simulink model "Dc_motor_Rpi"  (R2019a)
settings: Solver=FixedStepAuto  StartTime=0.0  StopTime=inf  FixedStep=0.02  RelTol=1e-3  EnableMultiTasking=on
libraries: embdlinuxlib x2, raspberrypilib x2
settings Model: SimulationMode=external  Creator=Ghofrane  LastModifiedBy=Ghofrane
settings SolverCC: PositivePriorityOrder=on
settings OptimizationCC: EnhancedBackFolding=on  PassReuseOutputArgsAs=Individual arguments  MaxStackSize=64  OptimizeBlockOrder=speed  DifferentSizesBufferReuse=on  OptimizationCustomize=off
settings DebuggingCC: ParameterTunabilityLossMsg=error
settings HardwareCC: ProdBitPerPointer=32  ProdBitPerSizeT=32  ProdBitPerPtrDiffT=32  ProdLargestAtomicInteger=Long  ProdLargestAtomicFloat=Double  ProdWordSize=32  ProdLongLongMode=on  ProdHWDeviceType=ARM Compatible->ARM Cortex
settings SFSimCC: MATLABDynamicMemAlloc=off
settings RTWCC: SystemTargetFile=ert.tlc  HardwareBoard=Raspberry Pi  TLCOptions="-aInlineSetEventsForThisBaseRateFcn=TLC_FALSE -aSuppressMultiTaskScheduler=TLC_FALSE  -aRateBasedStepFcn=0"  TemplateMakefile=ert_default_tmf  GenerateReport=on  Toolchain=GNU GCC Raspberry Pi  BuildConfiguration=Faster Runs  IncludeHyperlinkInReport=on  LaunchReport=on  GenerateTraceInfo=on  GenerateTraceReport=on  GenerateTraceReportSl=on  GenerateTraceReportSf=on  GenerateTraceReportEml=on
settings CodeAppCC: ForceParamTrailComments=on  IgnoreCustomStorageClasses=off  OperatorAnnotations=on  SimulinkDataObjDesc=on  SFDataObjDesc=on  InsertBlockDesc=on
settings ERTTargetCC: SupportVariableSizeSignals=on

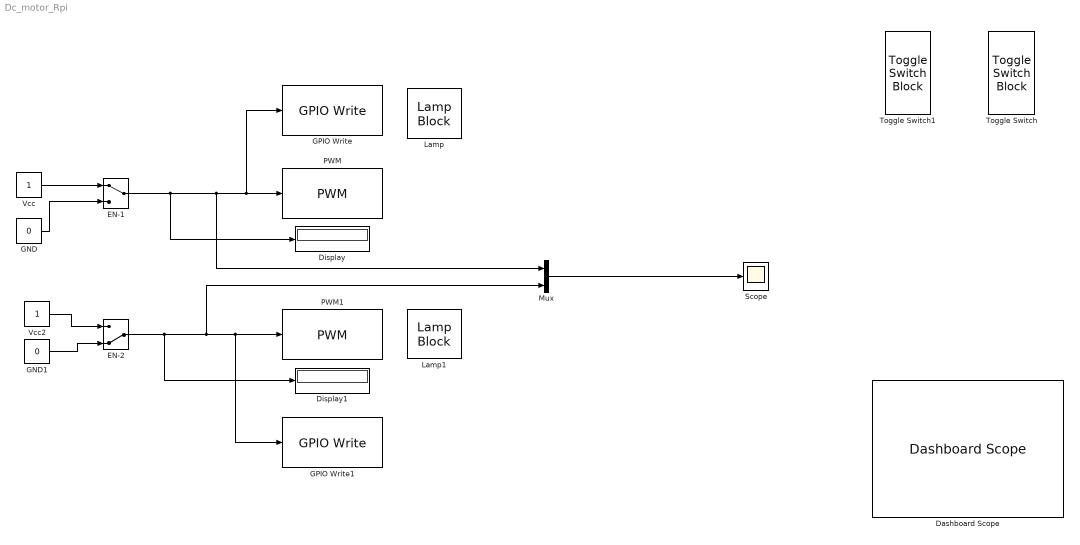
== system Dc_motor_Rpi ==
  Dashboard Scope : DashboardScope
  Display : Display
  Display1 : Display
  EN-1 : ManualSwitch
  EN-2 : ManualSwitch  CurrentSetting=0
  GND : Constant  Value=0
  "GND1 " : Constant  Value=0
  GPIO Write : embdlinuxlib/GPIO Write  board=Pi 2 Model B  gpio=19  direction=Output  blockPlatform=Raspberry Pi
      settings: SourceProductName=Simulink Coder Support Package for BeagleBone Blue Hardware  SourceProductBaseCode=SC_BEAGLEBONE_BLUE
  GPIO Write1 : embdlinuxlib/GPIO Write  board=Pi 2 Model B  gpio=26  direction=Output  blockPlatform=Raspberry Pi
      settings: SourceProductName=Simulink Coder Support Package for BeagleBone Blue Hardware  SourceProductBaseCode=SC_BEAGLEBONE_BLUE
  Lamp : LampBlock
  Lamp1 : LampBlock
  Mux : Mux  Inputs=2
  PWM : raspberrypilib/PWM  board=Pi 2 Model B  Pin_=21  Frequency=500  blockPlatform=Raspberry Pi
      settings: SourceProductName=Simulink Support Package for Raspberry Pi Hardware  SourceProductBaseCode=RASPPI
  PWM1 : raspberrypilib/PWM  board=Pi 2 Model B  Pin_=20  Frequency=500  blockPlatform=Raspberry Pi
      settings: SourceProductName=Simulink Support Package for Raspberry Pi Hardware  SourceProductBaseCode=RASPPI
  Scope : Scope
  Toggle Switch : ToggleSwitchBlock
      settings: Values={{'Off', 'On'}, [0 1]}
  Toggle Switch1 : ToggleSwitchBlock
      settings: Values={{'Off', 'On'}, [0 1]}
  Vcc : Constant
  Vcc2 : Constant
  wires:
  Vcc/1 -> EN-1/1
  EN-1/1 -> Display/1, Mux/1, GPIO Write/1, PWM/1
  GND/1 -> EN-1/2
  Vcc2/1 -> EN-2/1
  "GND1 "/1 -> EN-2/2
  EN-2/1 -> Display1/1, Mux/2, GPIO Write1/1, PWM1/1
  Mux/1 -> Scope/1
